simulink model "Single_Phase_Inverter_B2"  (R2016b)
settings: Solver=ode45  StartTime=0.0  StopTime=1  RelTol=1e-3  EnableMultiTasking=on
libraries: powerlib x18, dspstat3 x6, powerlib_meascontrol x1
settings Model: Creator=Rangga  LastModifiedBy=Rangga Putra
settings OptimizationCC: LifeSpan=inf
settings DebuggingCC: SFUnexpectedBacktrackingDiag=warning  SFNoUnconditionalDefaultTransitionDiag=warning  SFExecutionAtInitializationDiag=none
settings HardwareCC: ProdBitPerSizeT=32  ProdBitPerPtrDiffT=32  ProdWordSize=32  ProdHWDeviceType=Specified
settings GRTTargetCC: TargetLangStandard=C89/C90 (ANSI)  GeneratePreprocessorConditionals=Disable all
settings ConfigComp: CovMetricSettings=dw  CovHtmlReporting=on  CovSaveCumulativeToWorkspaceVar=on  CovSaveSingleToWorkspaceVar=on  CovExternalEMLEnable=off

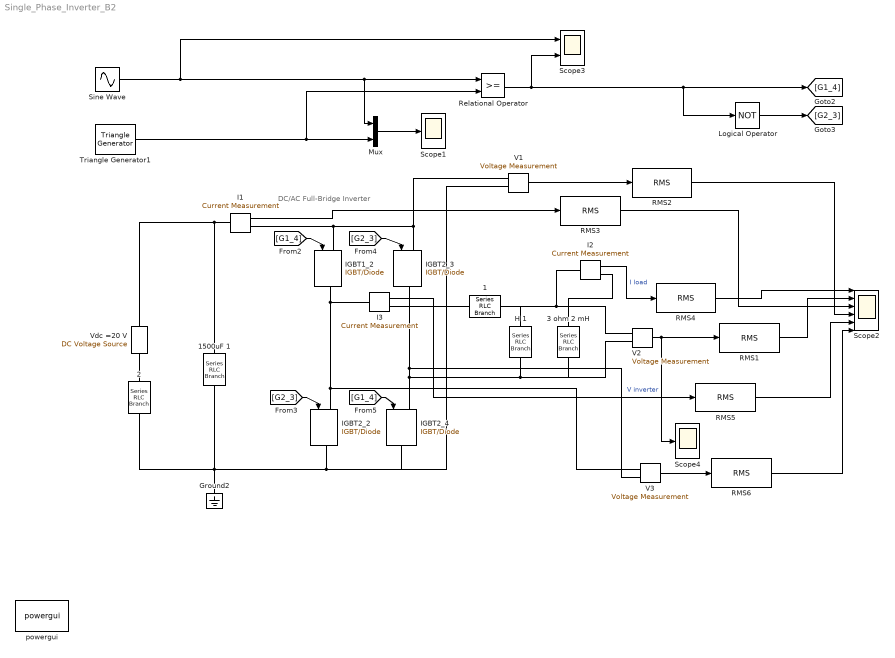
== system Single_Phase_Inverter_B2 ==
  note: DC/AC Full-Bridge Inverter
  " 1" : powerlib/Elements/Series RLC Branch  LConnTagsString=__new0  RConnTagsString=__new0  BranchType=L  Resistance=3  Inductance=1000e-6  SetiL0=off  InitialCurrent=0  Capacitance=[]  Setx0=off  InitialVoltage=0  Measurements=None
  " 2" : powerlib/Elements/Series RLC Branch  LConnTagsString=__new0  RConnTagsString=__new0  BranchType=R  Resistance=1  Inductance=2e-3  SetiL0=off  InitialCurrent=0  Capacitance=0.0015  Setx0=off  InitialVoltage=0  Measurements=None
  1500uF 1 : powerlib/Elements/Series RLC Branch  LConnTagsString=__new0  RConnTagsString=__new0  BranchType=C  Resistance=3  Inductance=2e-3  SetiL0=off  InitialCurrent=0  Capacitance=4700e-6  Setx0=off  InitialVoltage=0  Measurements=None
  "3 ohm 2 mH " : powerlib/Elements/Series RLC Branch  LConnTagsString=__new0  RConnTagsString=__new0  BranchType=RL  Resistance=1  Inductance=2e-3  SetiL0=off  InitialCurrent=0  Capacitance=[]  Setx0=off  InitialVoltage=0  Measurements=None
  Ground2 : powerlib/Elements/Ground  LConnTagsString=a
  H 1 : powerlib/Elements/Series RLC Branch  LConnTagsString=__new0  RConnTagsString=__new0  BranchType=C  Resistance=3  Inductance=2e-3  SetiL0=off  InitialCurrent=0  Capacitance=10e-6  Setx0=off  InitialVoltage=0  Measurements=None
  I1 : powerlib/Measurements/Current Measurement  Tag=PoWeRsYsTeMmEaSuReMeNt  PhasorSimulation=off  OutputType=Magnitude  PSBequivalent=0
  I2 : powerlib/Measurements/Current Measurement  Tag=PoWeRsYsTeMmEaSuReMeNt  PhasorSimulation=off  OutputType=Magnitude  PSBequivalent=0
  I3 : powerlib/Measurements/Current Measurement  Tag=PoWeRsYsTeMmEaSuReMeNt  PhasorSimulation=off  OutputType=Magnitude  PSBequivalent=0
  IGBT1_2 : powerlib/Power Electronics/IGBT//Diode  Ron=1e-3  Rs=1e5  Cs=inf  Measurements=off
  IGBT2_2 : powerlib/Power Electronics/IGBT//Diode  Ron=1e-3  Rs=1e5  Cs=inf  Measurements=off
  IGBT2_3 : powerlib/Power Electronics/IGBT//Diode  Ron=1e-3  Rs=1e5  Cs=inf  Measurements=off
  IGBT2_4 : powerlib/Power Electronics/IGBT//Diode  Ron=1e-3  Rs=1e5  Cs=inf  Measurements=off
  Logical Operator : Logic  Operator=NOT  AllPortsSameDT=off  OutDataTypeStr=boolean
  Mux : Mux  Inputs=2
  RMS{1..6} (6 alike) : dspstat3/RMS  run=on  directionMode=Each column  dimension=1  InputProcessing=Columns as channels (frame based)  reset_popup=None
  Relational Operator : RelationalOperator  OutDataTypeStr=boolean  RndMeth=Nearest
  Scope1 : Scope
  Scope2 : Scope  NumInputPorts=6
  Scope3 : Scope  NumInputPorts=2
  Scope4 : Scope
  Sine Wave : Sin  Amplitude=.5  Frequency=2*pi*60  SampleTime=0
  Triangle Generator1 : powerlib_meascontrol/Pulse & Signal Generators/Triangle Generator  Freq=10000  Phase=0  Ts=0
  V1 : powerlib/Measurements/Voltage Measurement  Tag=PoWeRsYsTeMmEaSuReMeNt  PhasorSimulation=off  OutputType=Magnitude  PSBequivalent=0
  V2 : powerlib/Measurements/Voltage Measurement  Tag=PoWeRsYsTeMmEaSuReMeNt  PhasorSimulation=off  OutputType=Magnitude  PSBequivalent=0
  V3 : powerlib/Measurements/Voltage Measurement  Tag=PoWeRsYsTeMmEaSuReMeNt  PhasorSimulation=off  OutputType=Magnitude  PSBequivalent=0
  Vdc =20 V : powerlib/Electrical Sources/DC Voltage Source  Description=source block  Amplitude=20  Measurements=None
      settings: AttributesFormatString=\n
  powergui : powerlib/powergui  Priority=1  SimulationMode=Discrete  SolverType=Tustin/Backward Euler (TBE)  SampleTime=1e-6  frequency=60  SPID=on  DisableSnubberDevices=off  DisableRonSwitches=off  DisableVfSwitches=off  SwTol=0  DisplayEquations=off  Interpol=off  ExternalGateDelay=off  methode=off  Ts=10  FunctionMessages=off  echomessages=off  HookPort=off  EnableUseOfTLC=off  x0status=blocks  frequencyindice=0  Pbase=100e6  ErrMax=1e-4  Iterations=50  UnitsV=kV  UnitsW=MW  buscounter=0  RestoreLinks=warning  ResistiveCurrentMeasurement=off  Frange=[0:2:500]  Ylog=off  Xlog=on  ShowGrid=off  save=off  variable=ZData  structure=ScopeData  ZoomFFT=off  StartTime=0.2  cycles=2  DisplayStyle=2  fundamental=60  FreqAxis=off  MaxFrequency=1000  frequencyindicesteady=1  RmsSteady=1  display=off
  wires:
  I2/1 -> RMS4/1  "I load"
  [G1_4] -> IGBT1_2/1
  [G2_3] -> IGBT2_2/1
  [G2_3] -> IGBT2_3/1
  [G1_4] -> IGBT2_4/1
  Sine Wave/1 -> Scope3/1, Mux/1, Relational Operator/1
  Relational Operator/1 -> Scope3/2, Logical Operator/1, [G1_4]
  Logical Operator/1 -> [G2_3]
  Triangle Generator1/1 -> Mux/2, Relational Operator/2
  Mux/1 -> Scope1/1
  V2/1 -> Scope4/1, RMS1/1  "V inverter"
  V1/1 -> RMS2/1
  I1/1 -> RMS3/1
  RMS2/1 -> Scope2/4
  RMS3/1 -> Scope2/3
  RMS1/1 -> Scope2/2
  RMS4/1 -> Scope2/1
  I3/1 -> RMS5/1
  RMS5/1 -> Scope2/5
  V3/1 -> RMS6/1
  RMS6/1 -> Scope2/6
  connections:
  " 1"/LConn1 -- H 1/LConn1 -- I2/LConn1 -- V2/LConn1
  V1/LConn2 -- IGBT2_4/RConn1 -- IGBT2_2/RConn1 -- 1500uF 1/RConn1 -- " 2"/RConn1 -- Ground2/LConn1
  IGBT1_2/LConn1 -- I1/RConn1 -- IGBT2_3/LConn1 -- V1/LConn1
  IGBT1_2/RConn1 -- I3/LConn1 -- V3/LConn1 -- IGBT2_2/LConn1
  IGBT2_3/RConn1 -- V3/LConn2 -- H 1/RConn1 -- V2/LConn2 -- "3 ohm 2 mH "/RConn1 -- IGBT2_4/LConn1
  " 2"/LConn1 -- Vdc =20 V/LConn1
  I1/LConn1 -- Vdc =20 V/RConn1 -- 1500uF 1/LConn1
  "3 ohm 2 mH "/LConn1 -- I2/RConn1
  I3/RConn1 -- " 1"/RConn1
